simulink model "DIM_DisplayMode_A3"  (R2022b)
settings: configuration reference "CommonModelConfiguration" (kept outside this file)
undefined symbols (not defined in the file): cc_param_100, cc_param_223
settings Model: Creator=vnarayan  LastModifiedBy=AJOSHI11
settings ConfigSetRef: SourceName=CommonModelConfiguration  SourceLocation=Base Workspace

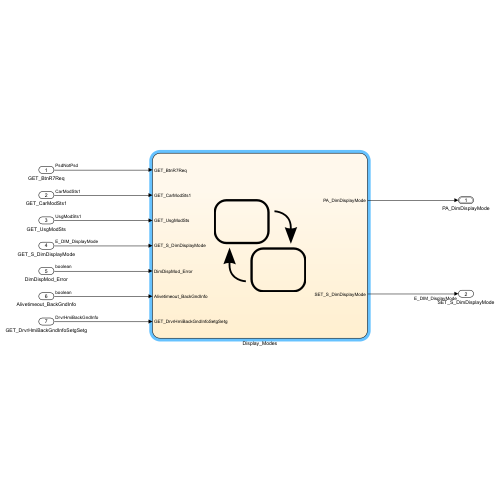
[thumbnail: Simulink's stored preview of the top-level diagram]
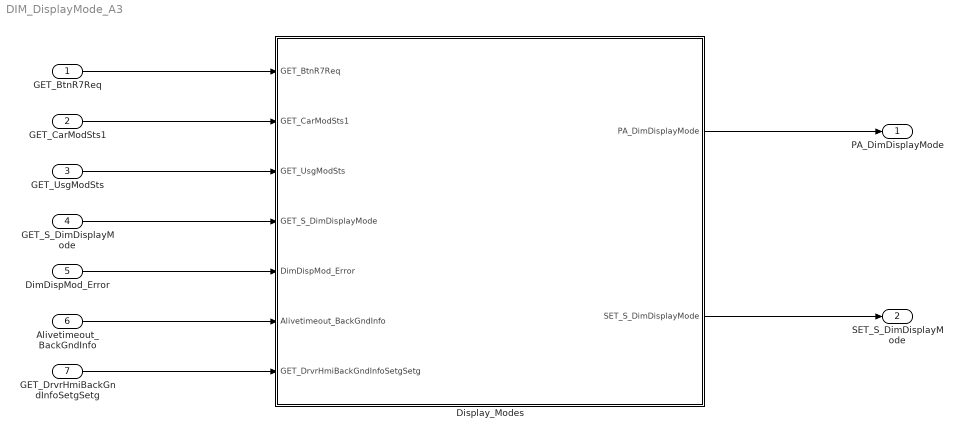
== system DIM_DisplayMode_A3 ==
  GET_BtnR7Req : Inport  OutDataTypeStr=Enum: PsdNotPsd
  GET_CarModSts1 : Inport  Port=2  OutDataTypeStr=Enum: CarModSts1
  GET_UsgModSts : Inport  Port=3  OutDataTypeStr=Enum: UsgModSts1
  GET_S_DimDisplayMode : Inport  Port=4  OutDataTypeStr=Enum: E_DIM_DisplayMode
  DimDispMod_Error : Inport  Port=5  OutDataTypeStr=boolean
  Alivetimeout_BackGndInfo : Inport  Port=6  OutDataTypeStr=boolean
  GET_DrvrHmiBackGndInfoSetgSetg : Inport  Port=7  OutDataTypeStr=Enum: DrvrHmiBackGndInfo
  Display_Modes : Stateflow chart  TreatAsAtomicUnit=on
  PA_DimDisplayMode : Outport  OutDataTypeStr=Bus: PA_StatusAndDisplayMode  VectorParamsAs1DForOutWhenUnconnected=off
  SET_S_DimDisplayMode : Outport  Port=2  OutDataTypeStr=Enum: E_DIM_DisplayMode  VectorParamsAs1DForOutWhenUnconnected=off
  wires:
  GET_CarModSts1/1 -> Display_Modes/2(GET_CarModSts1)
  GET_BtnR7Req/1 -> Display_Modes/1(GET_BtnR7Req)
  GET_S_DimDisplayMode/1 -> Display_Modes/4(GET_S_DimDisplayMode)
  GET_UsgModSts/1 -> Display_Modes/3(GET_UsgModSts)
  Display_Modes/1(PA_DimDisplayMode) -> PA_DimDisplayMode/1
  Display_Modes/2(SET_S_DimDisplayMode) -> SET_S_DimDisplayMode/1
  DimDispMod_Error/1 -> Display_Modes/5(DimDispMod_Error)
  Alivetimeout_BackGndInfo/1 -> Display_Modes/6(Alivetimeout_BackGndInfo)
  GET_DrvrHmiBackGndInfoSetgSetg/1 -> Display_Modes/7(GET_DrvrHmiBackGndInfoSetgSetg)

== stateflow chart DIM_DisplayMode_A3/Display_Modes ==
  state isActive = activationCheck [function]
    (default) -> (junction 247)
    (junction 247) -> (junction 248) [order 1] : % Activation conditions
        | [GET_CarModSts1==CarModSts1.CarModSts1_CarModNorm &&...
        | (GET_UsgModSts==UsgModSts1.UsgModSts1_UsgModDrvg ||...
        | GET_UsgModSts==UsgModSts1.UsgModSts1_UsgModActv)]
    (junction 247) -> (junction 249) [order 2] : {isActive = false;}
    (junction 248) -> (junction 250) : {isActive = true;}
    (junction 250) -> (junction 249)
    (junction 249) -> (junction 270)
  state SYSTEM_OK
    note: 
    state NO_DISPLAYMODE
      en:
      PA_DimDisplayMode = E_CommonStatus.NotPresent;
      SET_S_DimDisplayMode = E_DIM_DisplayMode.Calm;
    state DISPLAYMODE
      entry:
      PA_DimDisplayMode.Status = E_CommonStatus.Available;
      en, du:
      SET_S_DimDisplayMode = PA_DimDisplayMode.DisplayMode;
      state button7pushed [function]
        (default) -> (junction 422)
        (junction 422) -> (junction 423) [order 1] : [hasChangedTo(GET_BtnR7Req,PsdNotPsd.PsdNotPsd_Psd)]
        (junction 422) -> (junction 424) [order 2] : {button7pushed = false}
        (junction 423) -> (junction 425) : {button7pushed = true}
        (junction 425) -> (junction 424)
        (junction 424) -> (junction 426)
      state confNavi [function]
        (default) -> (junction 388)
        (junction 388) -> (junction 399) [order 1] : [cc_param_100~=3 &&...
            | cc_param_223>=3 &&...
            | (GET_DrvrHmiBackGndInfoSetgSetg~=DrvrHmiBackGndInfo.DrvrHmiBackGndInfoSetg1 ||...
            |  Alivetimeout_BackGndInfo)]
        (junction 388) -> (junction 401) [order 2] : {confNavi = false}
        (junction 399) -> (junction 400) : {confNavi = true}
        (junction 400) -> (junction 401)
        (junction 401) -> (junction 406)
      state confCarCentric [function]
        (default) -> (junction 410)
        (junction 410) -> (junction 411) [order 1] : [cc_param_100~=3 &&...
            | cc_param_223>=3 &&...
            | LCFG_DisplayMode_CarCentric &&...
            | cc_param_311 == 3]
        (junction 410) -> (junction 412) [order 2] : {confCC = false}
        (junction 411) -> (junction 413) : {confCC = true}
        (junction 413) -> (junction 412)
        (junction 412) -> (junction 414)
      state NAVI
        entry:
        PA_DimDisplayMode.DisplayMode = ...
        E_DIM_DisplayMode.Navi;
      state CALM
        entry:
        PA_DimDisplayMode.DisplayMode = ...
        E_DIM_DisplayMode.Calm;
      state SURROUND
        entry:
        PA_DimDisplayMode.DisplayMode = ...
        E_DIM_DisplayMode.CarCentric;
      (default) -> (junction 374)
      (junction 374) -> (junction 442) [order 1] : %Navi preselected
          | [confNavi &&...
          | GET_S_DimDisplayMode==...
          | E_DIM_DisplayMode.Navi]
      (junction 374) -> (junction 434) [order 2] : %Surround preselected
          | [confCarCentric &&...
          | GET_S_DimDisplayMode==...
          | E_DIM_DisplayMode.CarCentric]
      (junction 434) -> (junction 435)
      (junction 442) -> NAVI
      (junction 374) -> CALM [order 3]
      CALM -> NAVI [order 1] : %Navi available
          | [button7pushed && confNavi]
      NAVI -> CALM [order 2] : %No surround
          | [button7pushed && ~confCarCentric]
      NAVI -> (junction 444) [order 1] : %Surround available
          | [button7pushed && confCarCentric]
      CALM -> SURROUND [order 2] : %Surround selected but not
          | %navi available
          | [button7pushed &&...
          | confCarCentric && ~confNavi]
      SURROUND -> CALM : [button7pushed]
      (junction 435) -> SURROUND
      (junction 444) -> SURROUND
    (default) -> (junction 183)
    (junction 183) -> NO_DISPLAYMODE [order 1] : [~activationCheck()]
    (junction 183) -> (junction 182) [order 2]
    NO_DISPLAYMODE -> DISPLAYMODE : [activationCheck()]
    DISPLAYMODE -> NO_DISPLAYMODE : [~activationCheck()]
    (junction 182) -> DISPLAYMODE
  state SYSTEM_ERROR
    entry:
    PA_DimDisplayMode.Status = E_CommonStatus.SystemError;
    note: 
    state No_DisplayMode
    state DisplayMode
      DisplayMode -> (junction 360) [order 1]
      (junction 360) -> (junction 359) [order 1] : [cc_param_100==3]
      (junction 360) -> (junction 358) [order 2] : {PA_DimDisplayMode.DisplayMode = GET_S_DimDisplayMode;}
      (junction 359) -> (junction 364) : {PA_DimDisplayMode.DisplayMode  = E_DIM_DisplayMode.Calm;}
      (junction 364) -> (junction 358)
      (junction 358) -> (junction 361)
    (default) -> (junction 352)
    (junction 352) -> No_DisplayMode [order 1] : [~activationCheck()]
    (junction 352) -> (junction 353) [order 2]
    No_DisplayMode -> DisplayMode : [activationCheck()]
    DisplayMode -> No_DisplayMode [order 1] : [~activationCheck()]
    (junction 353) -> DisplayMode
  (default) -> (junction 242) : %The R7 button press is applicable in
      | %this logic only when the AppMenu is closed
  (junction 242) -> SYSTEM_OK [order 1] : [DimDispMod_Error==false]
  (junction 242) -> (junction 175) [order 2]
  SYSTEM_ERROR -> SYSTEM_OK : %If no system error is active then the
      | %function return to the system ok state
      |  [DimDispMod_Error==false]
  SYSTEM_OK -> SYSTEM_ERROR : %If there is a system error then the
      | %function enters an Error State
      |  [DimDispMod_Error==true]
  (junction 175) -> SYSTEM_ERROR
  data: isActive function_output boolean; GET_BtnR7Req input Enum: PsdNotPsd; PA_DimDisplayMode output Bus: PA_StatusAndDisplayMode; GET_CarModSts1 input Enum: CarModSts1; GET_UsgModSts input Enum: UsgModSts1; GET_S_DimDisplayMode input Enum: E_DIM_DisplayMode; SET_S_DimDisplayMode output Enum: E_DIM_DisplayMode; DimDispMod_Error input boolean; cc_param_100 parameter; cc_param_223 parameter; Alivetimeout_BackGndInfo input boolean; GET_DrvrHmiBackGndInfoSetgSetg input Enum: DrvrHmiBackGndInfo
